simulink model "RLC_Sim_2013b"  (Simulink 8.2)
settings: Solver=ode45  SolverMode=SingleTasking  StartTime=0.0  StopTime=10.0  RelTol=1e-3
values from neighbouring files (symbols this model uses):
  C = 1    [RLC_Parameters.m]
  L = 1    [RLC_Parameters.m]
  R = 2    [RLC_Parameters.m]
  v = 5    [RLC_Parameters.m]
settings Model: Creator=Sergio  LastModifiedBy=Sergio  CovMetricSettings=dwe  CovHtmlReporting=off  covSaveCumulativeToWorkspaceVar=off  CovSaveSingleToWorkspaceVar=off  CovExternalEMLEnable=on
settings DataIOCC: LimitDataPoints=off  SaveFormat=StructureWithTime  SignalLoggingSaveFormat=Dataset
settings OptimizationCC: ExpressionDepthLimit=128
settings DebuggingCC: UnderspecifiedInitializationDetection=Simplified  MergeDetectMultiDrivingBlocksExec=error  SolverPrmCheckMsg=none  FcnCallInpInsideContextMsg=EnableAllAsError  FrameProcessingCompatibilityMsg=error  StateNameClashWarn=none  SFUnexpectedBacktrackingDiag=error  SFNoUnconditionalDefaultTransitionDiag=error
settings HardwareCC: ProdBitPerPointer=64  ProdLargestAtomicFloat=Float  ProdIntDivRoundTo=Zero  ProdEndianess=LittleEndian  ProdHWDeviceType=Specified
settings ModelReferenceCC: PropagateSignalLabelsOutOfModel=on
settings GRTTargetCC: CodeReplacementLibrary=C99 (ISO)  GeneratePreprocessorConditionals=Use local settings  CombineOutputUpdateFcns=on  GRTInterface=off

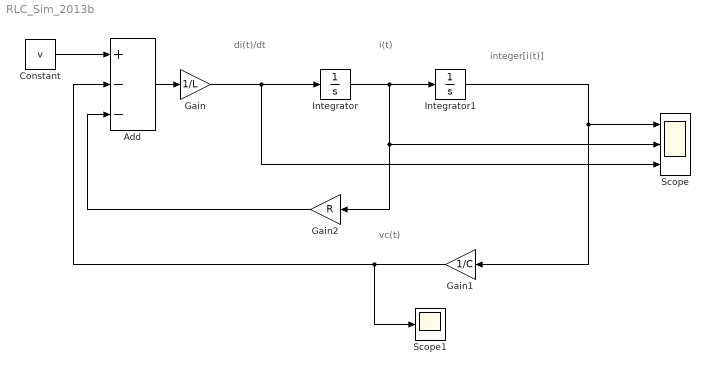
== system RLC_Sim_2013b ==
  note: di(t)/dt
  note: i(t)
  note: integer[i(t)]
  note: vc(t)
  Add : Sum  Inputs=+--
  Constant : Constant  Value=v
  Gain : Gain  Gain=1/L
  Gain1 : Gain  Gain=1/C
  Gain2 : Gain  Gain=R
  Integrator : Integrator
  Integrator1 : Integrator
  Scope : Scope  NumInputPorts=3
      settings: TimeRange=auto  MaxDataPoints=5000  SaveToWorkspace=off  SaveName=ScopeData  YMin=-1.38554~-1.38554~-1.38554  YMax=5.7095~5.7095~5.7095  SampleTime=-1
  Scope1 : Scope
      settings: TimeRange=auto  MaxDataPoints=5000  SaveToWorkspace=off  YMin=-0.62469  YMax=5.62219  SampleTime=-1
  wires:
  Gain/1 -> Scope/3, Integrator/1
  Integrator/1 -> Scope/2, Gain2/1, Integrator1/1
  Integrator1/1 -> Scope/1, Gain1/1
  Constant/1 -> Add/1
  Gain2/1 -> Add/3
  Gain1/1 -> Scope1/1, Add/2
  Add/1 -> Gain/1
